simulink model "FLANFIS"  (R2017b)
settings: Solver=FixedStepAuto  StartTime=0.0  StopTime=0.1  MaxStep=1e-4  RelTol=1e-3
libraries: powerlib x86, fl_lib x45, nesl_utility x9, powerlib_meascontrol x9, elec_lib x8, fuzblock x2, simulink x2
settings Model: Creator=wolfm  LastModifiedBy=wolfm

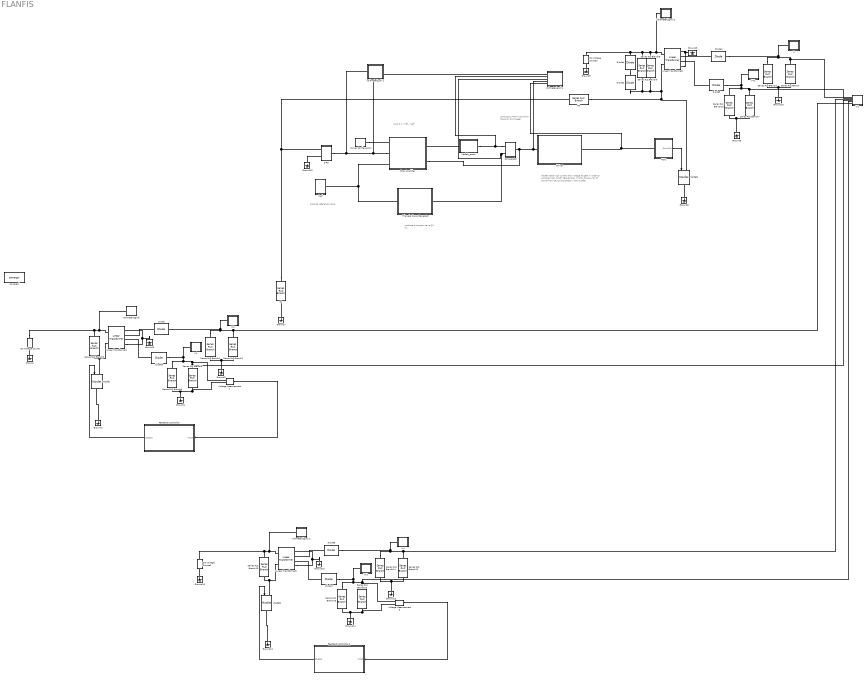
== system FLANFIS ==
  note: produces a PWM wave from the error and trigger
  note: Vout = A *( FB - Vref )
  note: produce a triangle wave @ f Hz
  note: produce reference Value
  note: Mosfet need high current and voltage at gate in order to produce high switch frequencies. IT also saves a lot of power from being dissipated in the mosfet.
  "Comparator " : Subsystem
  DC Voltage Source : powerlib/Electrical Sources/DC Voltage Source  Amplitude=24  Measurements=None
  DC Voltage Source1 : powerlib/Electrical Sources/DC Voltage Source  Amplitude=24  Measurements=None
  DC Voltage Source2 : powerlib/Electrical Sources/DC Voltage Source  Amplitude=24  Measurements=None
  Diode{,1..3,5..7} (7 alike) : powerlib/Power Electronics/Diode  Ron=0.001  Lon=0  Vf=0.7  IC=0  UseSnubber=0  Rs=500  Cs=250e-9  Measurements=off
  Diode4 : powerlib/Power Electronics/Diode  Ron=0.001  Lon=0  Vf=5.7  IC=0  UseSnubber=0  Rs=500  Cs=250e-9  Measurements=off
  Driver : Subsystem
  Error Amplifier : Subsystem
  "Feedback Controller " : Subsystem
  Feedback Controller 2 : Subsystem
  Ground{,1..16} (17 alike) : powerlib/Elements/Ground  LConnTagsString=a
  Linear Transformer1 : powerlib/Elements/Linear Transformer  UNITS=SI  NominalPower=[ 250e6 60 ]  winding1=[7.35e+05 4.3218 0.8]  winding2="[7.35e+05  4.3218 0.8]"  ThreeWindings=on  winding3=[7.35e+05 4.3218 0.8]  RmLm=[1.0805e+06 2880]  Measurements=None  DataType=on
  Linear Transformer2 : powerlib/Elements/Linear Transformer  UNITS=SI  NominalPower=[ 250e6 60 ]  winding1=[7.35e+05 4.3218 0.8]  winding2=[7.35e+05*15.5/24 4.3218 0.8]  ThreeWindings=on  winding3=[7.35e+05*15.5/24 4.3218 0.8]  RmLm=[1.0805e+06 2880]  Measurements=None  DataType=on
  Linear Transformer3 : powerlib/Elements/Linear Transformer  UNITS=SI  NominalPower=[ 250e6 60 ]  winding1=[7.35e+05 4.3218 0.8]  winding2="[7.35e+05  4.3218 0.8]"  ThreeWindings=on  winding3=[7.35e+05 4.3218 0.8]  RmLm=[1.0805e+06 2880]  Measurements=None  DataType=on
  Matlab_errors : Subsystem
  Mosfet : powerlib/Power Electronics/Mosfet  Ron=0.1  Lon=0  Rd=0.01  Vfd=0.7  IC=0  Rs=1e5  Cs=inf  Measurements=off
  Mosfet1 : powerlib/Power Electronics/Mosfet  Ron=0.1  Lon=0  Rd=0.01  Vfd=0.7  IC=0  Rs=1e5  Cs=inf  Measurements=off
  Mosfet2 : powerlib/Power Electronics/Mosfet  Ron=0.1  Lon=0  Rd=0.01  Vfd=0.7  IC=0  Rs=1e5  Cs=inf  Measurements=off
  PS-S : Subsystem
  R1 : powerlib/Elements/Series RLC Branch  LConnTagsString=__new0  RConnTagsString=__new0  BranchType=R  Resistance=3.9e+3  Inductance=0  SetiL0=off  InitialCurrent=0  Capacitance=0  Setx0=off  InitialVoltage=0  Measurements=None
  R5 : powerlib/Elements/Series RLC Branch  LConnTagsString=__new0  RConnTagsString=__new0  BranchType=R  Resistance=76.8e+3  Inductance=0  SetiL0=off  InitialCurrent=0  Capacitance=0  Setx0=off  InitialVoltage=0  Measurements=None
  S-PS : Subsystem
  Series RLC Branch{,2,5,7,12,15} (6 alike) : powerlib/Elements/Series RLC Branch  LConnTagsString=__new0  RConnTagsString=__new0  BranchType=R  Resistance=4.7e+3  Inductance=0  SetiL0=off  InitialCurrent=0  Capacitance=0  Setx0=off  InitialVoltage=0  Measurements=None
  Series RLC Branch{1,4,6,10,14,16} (6 alike) : powerlib/Elements/Series RLC Branch  LConnTagsString=__new0  RConnTagsString=__new0  BranchType=C  Resistance=15  Inductance=0  SetiL0=off  InitialCurrent=0  Capacitance=10e-6  Setx0=off  InitialVoltage=0  Measurements=None
  Series RLC Branch13 : powerlib/Elements/Series RLC Branch  LConnTagsString=__new0  RConnTagsString=__new0  BranchType=RC  Resistance=1e+3  Inductance=0  SetiL0=off  InitialCurrent=0  Capacitance=4.6e-7  Setx0=off  InitialVoltage=0  Measurements=None
  Series RLC Branch3 : powerlib/Elements/Series RLC Branch  LConnTagsString=__new0  RConnTagsString=__new0  BranchType=RC  Resistance=1e+3  Inductance=0  SetiL0=off  InitialCurrent=0  Capacitance=4.6e-6  Setx0=off  InitialVoltage=0  Measurements=None
  Series RLC Branch8 : powerlib/Elements/Series RLC Branch  LConnTagsString=__new0  RConnTagsString=__new0  BranchType=RC  Resistance=1e+3  Inductance=0  SetiL0=off  InitialCurrent=0  Capacitance=4.6e-6  Setx0=off  InitialVoltage=0  Measurements=None
  Series RLC Branch9 : powerlib/Elements/Series RLC Branch  LConnTagsString=__new0  RConnTagsString=__new0  BranchType=C  Resistance=15  Inductance=0  SetiL0=off  InitialCurrent=0  Capacitance=5.7e-6  Setx0=off  InitialVoltage=0  Measurements=None
  Solver Configuration : nesl_utility/Solver Configuration  PhysicalDomain=network_engine_domain  SubClassName=solver  LeftPortType=input  RightPortType=generic  Accelerate=off  Tones=[]  Harmonics=[]  SimulateNoise=off  Profile=off  UseLocalSampling=off  EnableSwitchedLinearOptims=on  FrequencyDomain=off  UseCCode=off  RelTol=0.001  AbsTol=1e-06  MinStep=1e-09  ToWorkspace=off  RevertToSquareIcSolve=off  NumHomotopyIterations=100  PhasorMode=off  PhasorModeNumHarmonics=1  DoDC=off  ResidualTolerance=1e-09  UseLocalSolver=off  LocalSolverChoice=NE_BACKWARD_EULER_ADVANCER  LocalSolverSampleTime=0.001  DoFixedCost=off  MaxNonlinIter=3  MaxModeIter=2  LinearAlgebra=Sparse  DelaysMemoryBudget=1024  AutomaticFiltering=on  FilteringTimeConstant=0.001
  Triangle Wave Generator : Subsystem
  V+ : Subsystem
  V+1 : Subsystem
  V+2 : Subsystem
  V- : Subsystem
  V-1 : Subsystem
  V-2 : Subsystem
  V-4 : Subsystem
  Voltage Measurement1 : powerlib/Measurements/Voltage Measurement  PhasorSimulation=off  OutputType=Complex  PSBequivalent=0
  Voltage Measurement3 : powerlib/Measurements/Voltage Measurement  PhasorSimulation=off  OutputType=Complex  PSBequivalent=0
  "Voltmeter(Sgnd) " : Subsystem
  Voltmeter(Sgnd) 1 : Subsystem
  Voltmeter(Sgnd) 2 : Subsystem
  Voltmeter(gnd) 1 : Subsystem
  Voltmeter(gnd) 4 : Subsystem
  Vref : Subsystem
  powergui : powerlib/powergui  Priority=1  SimulationMode=Discrete  SampleTime=50e-6  frequency=60  Iterations=50  frequencyindice=0  Pbase=100e6  ErrMax=1e-4  UnitsV=kV  UnitsW=MW  buscounter=0  FunctionMessages=off  echomessages=off  EnableUseOfTLC=off  CurrentSourceSwitches=off  DisableSnubberDevices=off  DisableRonSwitches=off  DisableVfSwitches=off  DisplayEquations=off  SolverType=Tustin/Backward Euler (TBE)  Interpol=off  ExternalGateDelay=off  methode=off  Ts=100  x0status=blocks  SPID=off  SwTol=0  HookPort=off  RestoreLinks=warning  ResistiveCurrentMeasurement=off  Frange=[0:2:500]  Ylog=off  Xlog=on  ShowGrid=off  save=off  variable=ZData  structure=0  ZoomFFT=off  StartTime=0.0  cycles=1  DisplayStyle=1  fundamental=60  FreqAxis=off  MaxFrequency=1000  frequencyindicesteady=1  RmsSteady=1  display=off
  wires:
  Voltage Measurement1/1 -> "Feedback Controller "/1("Input ")
  "Feedback Controller "/1("Output ") -> Mosfet/1
  Feedback Controller 2/1("Output ") -> Mosfet2/1
  Voltage Measurement3/1 -> Feedback Controller 2/1("Input ")
  PS-S/1("Simulink ") -> Mosfet1/1
  connections:
  Linear Transformer1/LConn2 -- Mosfet/LConn1 -- Series RLC Branch3/LConn1
  DC Voltage Source/RConn1 -- Series RLC Branch3/RConn1 -- Linear Transformer1/LConn1 -- "Voltmeter(Sgnd) "/LConn1
  Ground/LConn1 -- DC Voltage Source/LConn1
  Ground1/LConn1 -- Mosfet/RConn1
  Ground4/LConn1 -- Voltage Measurement1/LConn2 -- Series RLC Branch5/LConn1 -- Series RLC Branch6/LConn1
  Series RLC Branch5/RConn1 -- V-2/LConn4 -- Series RLC Branch6/RConn1 -- V+/LConn1 -- Diode3/RConn1 -- Voltage Measurement1/LConn1
  Series RLC Branch2/LConn1 -- Series RLC Branch4/LConn1 -- Ground2/LConn1
  Series RLC Branch4/RConn1 -- V-2/LConn6 -- Series RLC Branch2/RConn1 -- V-1/LConn1 -- Diode/LConn1
  Diode/RConn1 -- Linear Transformer1/RConn2
  Diode3/LConn1 -- Linear Transformer1/RConn3
  Linear Transformer1/RConn4 -- Ground3/LConn1 -- Linear Transformer1/RConn1
  Series RLC Branch13/LConn1 -- Linear Transformer3/LConn2 -- Mosfet2/LConn1
  Linear Transformer3/RConn1 -- Linear Transformer3/RConn4 -- Ground13/LConn1
  Series RLC Branch16/RConn1 -- Series RLC Branch15/RConn1 -- Voltage Measurement3/LConn1 -- V-2/LConn5 -- V+2/LConn1 -- Diode7/RConn1
  Series RLC Branch14/RConn1 -- Series RLC Branch12/RConn1 -- V-2/LConn3 -- V-4/LConn1 -- Diode6/LConn1
  Series RLC Branch16/LConn1 -- Ground14/LConn1 -- Voltage Measurement3/LConn2 -- Series RLC Branch15/LConn1
  Ground12/LConn1 -- Series RLC Branch12/LConn1 -- Series RLC Branch14/LConn1
  Voltmeter(Sgnd) 2/LConn1 -- Linear Transformer3/LConn1 -- DC Voltage Source2/RConn1 -- Series RLC Branch13/RConn1
  Ground11/LConn1 -- Mosfet2/RConn1
  Diode6/RConn1 -- Linear Transformer3/RConn2
  Ground10/LConn1 -- DC Voltage Source2/LConn1
  Diode7/LConn1 -- Linear Transformer3/RConn3
  Error Amplifier/LConn2 -- S-PS/RConn1 -- Voltmeter(gnd) 1/LConn1 -- Voltmeter(gnd) 4/LConn1
  Linear Transformer2/RConn1 -- Linear Transformer2/RConn4 -- Ground8/LConn1
  Driver/LConn1 -- Voltmeter(gnd) 4/LConn4 -- "Comparator "/RConn1 -- Error Amplifier/RConn2
  Series RLC Branch1/RConn1 -- V-2/LConn1 -- Series RLC Branch/RConn1 -- V-/LConn1 -- Diode1/LConn1
  R1/RConn1 -- R5/LConn1 -- S-PS/LConn1
  Series RLC Branch7/RConn1 -- V-2/LConn2 -- Series RLC Branch10/RConn1 -- V+1/LConn1 -- Diode5/RConn1
  Series RLC Branch10/LConn1 -- Series RLC Branch7/LConn1 -- Ground9/LConn1
  Voltmeter(gnd) 4/LConn5 -- PS-S/LConn1 -- Driver/RConn1
  R5/RConn1 -- Mosfet1/LConn1 -- Series RLC Branch8/LConn1 -- Series RLC Branch9/LConn1 -- Diode2/LConn1 -- Linear Transformer2/LConn2
  Vref/LConn1 -- Triangle Wave Generator/LConn1 -- Error Amplifier/LConn3
  Triangle Wave Generator/RConn1 -- "Comparator "/LConn2 -- Voltmeter(gnd) 4/LConn3
  Series RLC Branch9/RConn1 -- DC Voltage Source1/RConn1 -- Diode4/LConn1 -- Series RLC Branch8/RConn1 -- Linear Transformer2/LConn1 -- Voltmeter(Sgnd) 1/LConn1
  Series RLC Branch/LConn1 -- Series RLC Branch1/LConn1 -- Ground16/LConn1
  "Comparator "/LConn1 -- Matlab_errors/RConn1 -- Voltmeter(gnd) 4/LConn2
  Ground15/LConn1 -- S-PS/LConn2
  Ground5/LConn1 -- DC Voltage Source1/LConn1
  Ground6/LConn1 -- Mosfet1/RConn1
  Solver Configuration/RConn1 -- Error Amplifier/LConn1
  Diode4/RConn1 -- Diode2/RConn1
  Ground7/LConn1 -- R1/LConn1
  Matlab_errors/LConn1 -- Error Amplifier/RConn1
  Diode5/LConn1 -- Linear Transformer2/RConn3
  Diode1/RConn1 -- Linear Transformer2/RConn2

== system FLANFIS/Comparator  ==
  Comparator : elec_lib/Integrated Circuits/Comparator  V_OS=5 mV  V_OL=0 V  V_OH=5 V  C_IN=0 pF  R_OUT=2 Ohm  Delay=0 s
      settings: SourceProductName=Simscape Electronics  SourceProductBaseCode=SN
  Vin1 : PMIOPort  Port=1  Side=Left
  Output : PMIOPort  Port=2  Side=Right
  VIn2 : PMIOPort  Port=3  Side=Left
  connections:
  Vin1/RConn1 -- Comparator/LConn1
  Comparator/LConn2 -- VIn2/RConn1
  Comparator/RConn1 -- Output/RConn1

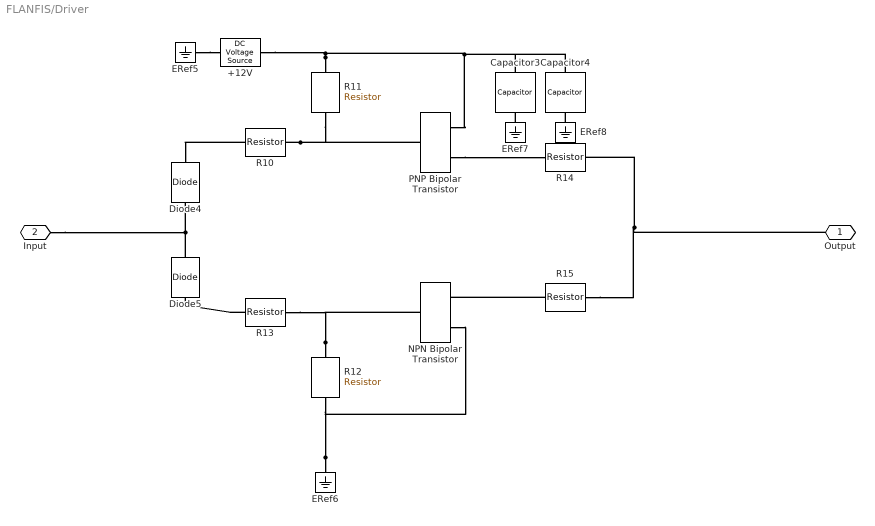
== system FLANFIS/Driver ==
  "+12V " : elec_lib/Additional Components/SPICE-Compatible Components/Sources/DC Voltage Source  DC=12 V
      settings: SourceProductName=Simscape Electronics  SourceProductBaseCode=SN
  Capacitor3 : fl_lib/Electrical/Electrical Elements/Capacitor  c=47e-6 F  r=0 Ohm  g=0 1/Ohm  i_specify=off  i_priority=None  i=0 A  i_nominal_specify=off  i_nominal_unit=A  i_nominal_value=1  v_specify=off  v_priority=None  v=0 V  v_nominal_specify=off  v_nominal_unit=V  v_nominal_value=1  vc_specify=off  vc_priority=High  vc=0 V  vc_nominal_specify=off  vc_nominal_unit=V  vc_nominal_value=1
  Capacitor4 : fl_lib/Electrical/Electrical Elements/Capacitor  c=100e-9 F  r=0 Ohm  g=0 1/Ohm  i_specify=off  i_priority=None  i=0 A  i_nominal_specify=off  i_nominal_unit=A  i_nominal_value=1  v_specify=off  v_priority=None  v=0 V  v_nominal_specify=off  v_nominal_unit=V  v_nominal_value=1  vc_specify=off  vc_priority=High  vc=0 V  vc_nominal_specify=off  vc_nominal_unit=V  vc_nominal_value=1
  Diode4 : elec_lib/Semiconductor Devices/Diode  ModelType=2  Vf=3.3 V  Ron=0.3 Ohm  Goff=1e-8 S  Rz=0.3 Ohm  Vz=50 V  C_PWL=5 pF  prmExp=1  I12=[.0137, .545] A  V12=[.6, .7] V  I1=0.0137 A  V1=0.6 V  IS=1e-12 A  ec=1  RS=0.01 Ohm  Tmeas=25 degC  BV=inf V  C_param=1  CJ0=5 pF  VJ=1 V  Mgrad=0.5  Vvec=[.1, 10, 100] V  Cvec=[3.5, 1, .4] pF  FC=0.5  Q_param=1  Irrm=-7.15 A  iF=4 A  didt=-750 A/us  trr=115 ns  TT=50 ns  tau=100 ns  T_param=1  IS_T2=1.25e-7 A  I1_T2=0.245 A  V1_T2=0.5 V  Tmeas2=125 degC  EG_param=1  EG=1.11 eV  XTI_param=1  XTI=3  dBVdT=0 V/K  Tdevice=25 degC  i_capacitor_specify=off  i_capacitor_priority=High  i_capacitor=0 A  i_capacitor_nominal_specify=off  i_capacitor_nominal_unit=A  i_capacitor_nominal_value=1  v_capacitor_specify=off  v_capacitor_priority=None  v_capacitor=0 V  v_capacitor_nominal_specify=off  v_capacitor_nominal_unit=V  v_capacitor_nominal_value=1  Rth=[0, 10] K/W  thermal_mass_parameterization=1  thermal_mass=[0, 1] J/K  thermal_time_constant=[0, 10] s  thermal_mass_initial_temperatures=[25, 25] degC
      settings: SourceProductName=Simscape Electronics  SourceProductBaseCode=SN
  Diode5 : elec_lib/Semiconductor Devices/Diode  ModelType=2  Vf=3.3 V  Ron=0.3 Ohm  Goff=1e-8 S  Rz=0.3 Ohm  Vz=50 V  C_PWL=5 pF  prmExp=1  I12=[.0137, .545] A  V12=[.6, .7] V  I1=0.0137 A  V1=0.6 V  IS=1e-12 A  ec=1  RS=0.01 Ohm  Tmeas=25 degC  BV=inf V  C_param=1  CJ0=5 pF  VJ=1 V  Mgrad=0.5  Vvec=[.1, 10, 100] V  Cvec=[3.5, 1, .4] pF  FC=0.5  Q_param=1  Irrm=-7.15 A  iF=4 A  didt=-750 A/us  trr=115 ns  TT=50 ns  tau=100 ns  T_param=1  IS_T2=1.25e-7 A  I1_T2=0.245 A  V1_T2=0.5 V  Tmeas2=125 degC  EG_param=1  EG=1.11 eV  XTI_param=1  XTI=3  dBVdT=0 V/K  Tdevice=25 degC  i_capacitor_specify=off  i_capacitor_priority=High  i_capacitor=0 A  i_capacitor_nominal_specify=off  i_capacitor_nominal_unit=A  i_capacitor_nominal_value=1  v_capacitor_specify=off  v_capacitor_priority=None  v_capacitor=0 V  v_capacitor_nominal_specify=off  v_capacitor_nominal_unit=V  v_capacitor_nominal_value=1  Rth=[0, 10] K/W  thermal_mass_parameterization=1  thermal_mass=[0, 1] J/K  thermal_time_constant=[0, 10] s  thermal_mass_initial_temperatures=[25, 25] degC
      settings: SourceProductName=Simscape Electronics  SourceProductBaseCode=SN
  ERef{5..8} (4 alike) : fl_lib/Electrical/Electrical Elements/Electrical Reference
  NPN Bipolar Transistor : elec_lib/Semiconductor Devices/NPN Bipolar Transistor  parameterization=1  prmDatasheet=1  prmEquCoeff=1  BF=100  IS=1e-14 A  ec=1  VAF=200 V  hfe=100  hoe=5e-5 1/Ohm  Ic_h=1 mA  Vce_h=5 V  V1=0.55 V  I1=0.5 mA  BR=1  Tmeas=25 degC  RC=0.01 Ohm  RE=1e-4 Ohm  RB=1 Ohm  C_BC=5 pF  C_BE=5 pF  TF=0 us  TR=0 us  hfe_T2=125  XTB=0  V1_T2=0.45 V  I1_T2=0.5 mA  Tmeas2=125 degC  EG=1.11 eV  XTI=3  TdeviceDatasheet=25 degC  TdeviceEquCoeff=25 degC  Rth=[ 0 10 ] K/W  thermal_mass_parameterization=1  thermal_mass=[ 0 1 ] J/K  thermal_time_constant=[ 0 10 ] s  thermal_mass_initial_temperatures=[ 25 25 ] degC
      settings: SourceProductName=Simscape Electronics  SourceProductBaseCode=SN
  PNP Bipolar Transistor : elec_lib/Semiconductor Devices/PNP Bipolar Transistor  parameterization=1  prmDatasheet=1  prmEquCoeff=1  BF=100  IS=1e-14 A  ec=1  VAF=200 V  hfe=100  hoe=5e-5 1/Ohm  Ic_h=-1 mA  Vce_h=-5 V  V1=-0.55 V  I1=-0.5 mA  BR=1  Tmeas=25 degC  RC=0.01 Ohm  RE=1e-4 Ohm  RB=1 Ohm  C_BC=5 pF  C_BE=5 pF  TF=0 us  TR=0 us  hfe_T2=125  XTB=0  V1_T2=-0.45 V  I1_T2=-0.5 mA  Tmeas2=125 degC  EG=1.11 eV  XTI=3  TdeviceDatasheet=25 degC  TdeviceEquCoeff=25 degC  Rth=[ 0 10 ] K/W  thermal_mass_parameterization=1  thermal_mass=[ 0 1 ] J/K  thermal_time_constant=[ 0 10 ] s  thermal_mass_initial_temperatures=[ 25 25 ] degC
      settings: SourceProductName=Simscape Electronics  SourceProductBaseCode=SN
  R10 : fl_lib/Electrical/Electrical Elements/Resistor  R=1e+3 Ohm  i_specify=off  i_priority=High  i=0 A  i_nominal_specify=off  i_nominal_unit=A  i_nominal_value=1  v_specify=off  v_priority=High  v=0 V  v_nominal_specify=off  v_nominal_unit=V  v_nominal_value=1
      settings: AttributesFormatString=%<R> %<R_unit>
  R11 : fl_lib/Electrical/Electrical Elements/Resistor  R=47e+3 Ohm  i_specify=off  i_priority=High  i=0 A  i_nominal_specify=off  i_nominal_unit=A  i_nominal_value=1  v_specify=off  v_priority=High  v=0 V  v_nominal_specify=off  v_nominal_unit=V  v_nominal_value=1
      settings: AttributesFormatString=%<R> %<R_unit>
  R12 : fl_lib/Electrical/Electrical Elements/Resistor  R=47e+3 Ohm  i_specify=off  i_priority=High  i=0 A  i_nominal_specify=off  i_nominal_unit=A  i_nominal_value=1  v_specify=off  v_priority=High  v=0 V  v_nominal_specify=off  v_nominal_unit=V  v_nominal_value=1
      settings: AttributesFormatString=%<R> %<R_unit>
  R13 : fl_lib/Electrical/Electrical Elements/Resistor  R=1e+3 Ohm  i_specify=off  i_priority=High  i=0 A  i_nominal_specify=off  i_nominal_unit=A  i_nominal_value=1  v_specify=off  v_priority=High  v=0 V  v_nominal_specify=off  v_nominal_unit=V  v_nominal_value=1
      settings: AttributesFormatString=%<R> %<R_unit>
  R14 : fl_lib/Electrical/Electrical Elements/Resistor  R=4.7 Ohm  i_specify=off  i_priority=High  i=0 A  i_nominal_specify=off  i_nominal_unit=A  i_nominal_value=1  v_specify=off  v_priority=High  v=0 V  v_nominal_specify=off  v_nominal_unit=V  v_nominal_value=1
      settings: AttributesFormatString=%<R> %<R_unit>
  R15 : fl_lib/Electrical/Electrical Elements/Resistor  R=4.7 Ohm  i_specify=off  i_priority=High  i=0 A  i_nominal_specify=off  i_nominal_unit=A  i_nominal_value=1  v_specify=off  v_priority=High  v=0 V  v_nominal_specify=off  v_nominal_unit=V  v_nominal_value=1
      settings: AttributesFormatString=%<R> %<R_unit>
  Output : PMIOPort  Port=1  Side=Right
  Input : PMIOPort  Port=2  Side=Left
  connections:
  Diode5/RConn1 -- Input/RConn1 -- Diode4/LConn1
  R15/RConn1 -- R14/LConn1 -- Output/RConn1
  ERef6/LConn1 -- R12/LConn1 -- NPN Bipolar Transistor/RConn2
  R11/RConn1 -- "+12V "/LConn1 -- Capacitor4/LConn1 -- Capacitor3/LConn1 -- PNP Bipolar Transistor/RConn1
  R12/RConn1 -- R13/LConn1 -- NPN Bipolar Transistor/LConn1
  PNP Bipolar Transistor/RConn2 -- R14/RConn1
  R15/LConn1 -- NPN Bipolar Transistor/RConn1
  R10/RConn1 -- Diode4/RConn1
  ERef5/LConn1 -- "+12V "/RConn1
  R13/RConn1 -- Diode5/LConn1
  ERef7/LConn1 -- Capacitor3/RConn1
  R10/LConn1 -- R11/LConn1 -- PNP Bipolar Transistor/LConn1
  ERef8/LConn1 -- Capacitor4/RConn1

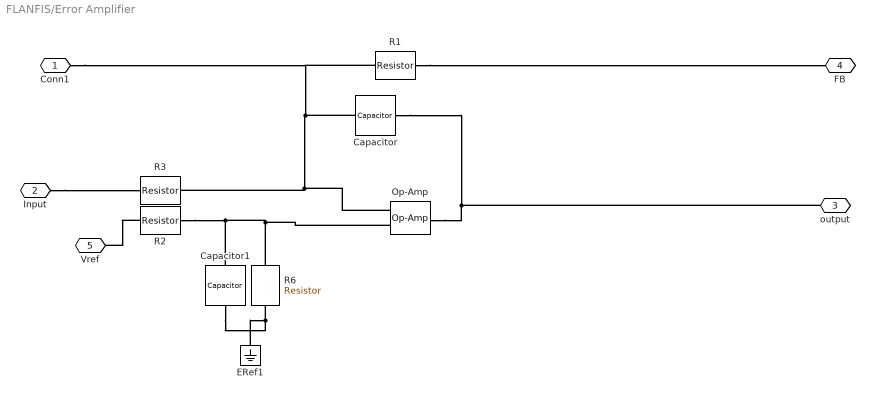
== system FLANFIS/Error Amplifier ==
  Capacitor : fl_lib/Electrical/Electrical Elements/Capacitor  c=100e-12 F  r=5 Ohm  g=0 1/Ohm  i_specify=off  i_priority=None  i=0 A  i_nominal_specify=off  i_nominal_unit=A  i_nominal_value=1  v_specify=off  v_priority=None  v=0 V  v_nominal_specify=off  v_nominal_unit=V  v_nominal_value=1  vc_specify=on  vc_priority=None  vc=0 V  vc_nominal_specify=off  vc_nominal_unit=V  vc_nominal_value=1
  Capacitor1 : fl_lib/Electrical/Electrical Elements/Capacitor  c=100e-12 F  r=0 Ohm  g=0 1/Ohm  i_specify=off  i_priority=None  i=0 A  i_nominal_specify=off  i_nominal_unit=A  i_nominal_value=1  v_specify=off  v_priority=None  v=0 V  v_nominal_specify=off  v_nominal_unit=V  v_nominal_value=1  vc_specify=off  vc_priority=High  vc=0 V  vc_nominal_specify=off  vc_nominal_unit=V  vc_nominal_value=1
  ERef1 : fl_lib/Electrical/Electrical Elements/Electrical Reference
  Op-Amp : fl_lib/Electrical/Electrical Elements/Op-Amp  outI_specify=off  outI_priority=None  outI=0 A  outI_nominal_specify=off  outI_nominal_unit=A  outI_nominal_value=1
  R{1..3,6} (4 alike) : fl_lib/Electrical/Electrical Elements/Resistor  R=10e3 Ohm  i_specify=off  i_priority=High  i=0 A  i_nominal_specify=off  i_nominal_unit=A  i_nominal_value=1  v_specify=off  v_priority=High  v=0 V  v_nominal_specify=off  v_nominal_unit=V  v_nominal_value=1
      settings: AttributesFormatString=%<R> %<R_unit>
  Conn1 : PMIOPort  Port=1  Side=Left
  Input : PMIOPort  Port=2  Side=Left
  "output " : PMIOPort  Port=3  Side=Right
  FB : PMIOPort  Port=4  Side=Right
  Vref : PMIOPort  Port=5  Side=Left
  connections:
  R1/RConn1 -- FB/RConn1
  R2/LConn1 -- Vref/RConn1
  Capacitor/LConn1 -- Op-Amp/LConn2 -- R3/RConn1 -- Conn1/RConn1 -- R1/LConn1
  R6/LConn1 -- Op-Amp/LConn1 -- R2/RConn1 -- Capacitor1/LConn1
  R6/RConn1 -- Capacitor1/RConn1 -- ERef1/LConn1
  Input/RConn1 -- R3/LConn1
  Capacitor/RConn1 -- "output "/RConn1 -- Op-Amp/RConn1

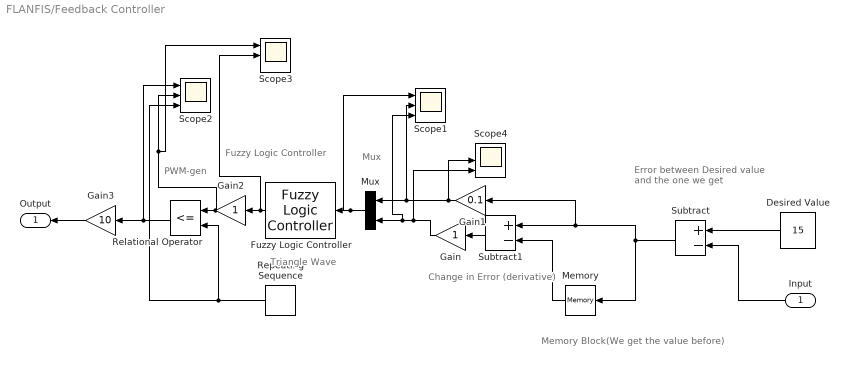
== system FLANFIS/Feedback Controller  ==
  note: PWM-gen
  note: Triangle Wave
  note: Fuzzy Logic Controller
  note: Mux
  note: Change in Error (derivative)
  note: Memory Block(We get the value before)
  note: Error between Desired value and the one we get
  "Input " : Inport
  Desired Value : Constant  Value=15
  Fuzzy Logic Controller : fuzblock/Fuzzy Logic  Controller  FIS='flc.fis'  OutputSampleNumber=1e+2  DataType=double  FuzzifiedInputs=off  RuleFiringStrengths=off  RuleOutputs=off  AggregatedOutputs=off  SimulateUsing=Interpreted execution
  Gain : Gain  OutMax=[15]
  Gain1 : Gain  Gain=0.1  OutMax=[15]
  Gain2 : Gain  OutMax=[15]
  Gain3 : Gain  Gain=10  OutMax=[15]
  Memory : Memory
  Mux : Mux  Inputs=2
  Relational Operator : RelationalOperator  Operator=<=  OutDataTypeStr=boolean  RndMeth=Simplest
  Repeating Sequence : simulink/Sources/Repeating Sequence  rep_seq_t=[0 0.5 1]/1000  rep_seq_y=[0 1 0]
  Scope{1..4} (4 alike) : Scope  NumInputPorts=3
  Subtract : Sum  Inputs=+-
  Subtract1 : Sum  Inputs=+-
  "Output " : Outport
  wires:
  Repeating Sequence/1 -> Scope2/3, Relational Operator/2
  Relational Operator/1 -> Scope2/1, Gain3/1
  Mux/1 -> Scope1/1, Fuzzy Logic Controller/1
  Subtract/1 -> Memory/1, Gain1/1, Subtract1/1
  Desired Value/1 -> Subtract/1
  "Input "/1 -> Subtract/2
  Memory/1 -> Subtract1/2
  Subtract1/1 -> Gain/1
  Gain/1 -> Scope4/3, Scope1/3, Mux/2
  Gain1/1 -> Scope4/2, Scope1/2, Mux/1
  Gain2/1 -> Scope3/1, Scope2/2, Relational Operator/1
  Fuzzy Logic Controller/1 -> Scope3/2, Gain2/1
  Gain3/1 -> "Output "/1

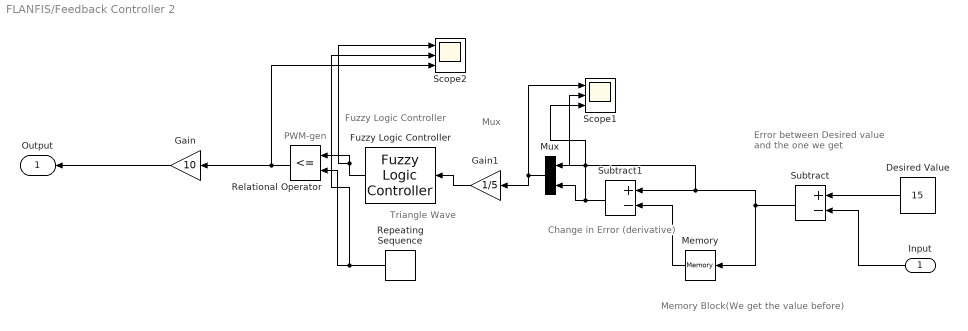
== system FLANFIS/Feedback Controller 2 ==
  note: PWM-gen
  note: Triangle Wave
  note: Fuzzy Logic Controller
  note: Mux
  note: Change in Error (derivative)
  note: Memory Block(We get the value before)
  note: Error between Desired value and the one we get
  "Input " : Inport
  Desired Value : Constant  Value=15
  Fuzzy Logic Controller : fuzblock/Fuzzy Logic  Controller  FIS='flc.fis'  OutputSampleNumber=101  DataType=double  FuzzifiedInputs=off  RuleFiringStrengths=off  RuleOutputs=off  AggregatedOutputs=off  SimulateUsing=Interpreted execution
  Gain : Gain  Gain=10
  Gain1 : Gain  Gain=1/5
  Memory : Memory
  Mux : Mux  Inputs=2
  Relational Operator : RelationalOperator  Operator=<=  OutDataTypeStr=boolean  RndMeth=Simplest
  Repeating Sequence : simulink/Sources/Repeating Sequence  rep_seq_t=[0 0.5 1]/500  rep_seq_y=[0 15 0]
  Scope1 : Scope  NumInputPorts=3
  Scope2 : Scope  NumInputPorts=3
  Subtract : Sum  Inputs=+-
  Subtract1 : Sum  Inputs=+-
  "Output " : Outport
  wires:
  Subtract1/1 -> Scope1/2, Scope1/3, Mux/2
  Repeating Sequence/1 -> Scope2/2, Relational Operator/2
  Relational Operator/1 -> Scope2/3, Gain/1
  Subtract/1 -> Memory/1, Mux/1, Subtract1/1
  Desired Value/1 -> Subtract/1
  "Input "/1 -> Subtract/2
  Memory/1 -> Subtract1/2
  Fuzzy Logic Controller/1 -> Scope2/1, Relational Operator/1
  Gain/1 -> "Output "/1
  Mux/1 -> Scope1/1, Gain1/1
  Gain1/1 -> Fuzzy Logic Controller/1

== system FLANFIS/Matlab_errors ==
  Capacitor5 : fl_lib/Electrical/Electrical Elements/Capacitor  c=100e-6 F  r=10 Ohm  g=0 1/Ohm  i_specify=off  i_priority=None  i=0 A  i_nominal_specify=off  i_nominal_unit=A  i_nominal_value=1  v_specify=off  v_priority=None  v=0 V  v_nominal_specify=off  v_nominal_unit=V  v_nominal_value=1  vc_specify=on  vc_priority=None  vc=0 V  vc_nominal_specify=off  vc_nominal_unit=V  vc_nominal_value=1
  ERef4 : fl_lib/Electrical/Electrical Elements/Electrical Reference
  R7 : fl_lib/Electrical/Electrical Elements/Resistor  R=10e5 Ohm  i_specify=off  i_priority=High  i=0 A  i_nominal_specify=off  i_nominal_unit=A  i_nominal_value=1  v_specify=off  v_priority=High  v=0 V  v_nominal_specify=off  v_nominal_unit=V  v_nominal_value=1
      settings: AttributesFormatString=%<R> %<R_unit>
  Output : PMIOPort  Port=1  Side=Right
  "Input " : PMIOPort  Port=2  Side=Left
  connections:
  R7/LConn1 -- "Input "/RConn1
  ERef4/LConn1 -- Capacitor5/RConn1
  R7/RConn1 -- Output/RConn1 -- Capacitor5/LConn1

== system FLANFIS/PS-S ==
  ERef9 : fl_lib/Electrical/Electrical Elements/Electrical Reference
  PS-Simulink Converter1 : nesl_utility/PS-Simulink Converter  PhysicalDomain=network_engine_domain  SubClassName=ps_output  LeftPortType=input  RightPortType=output  PseudoPeriodic=off  Frequencies=[]  Unit=1  AffineConversion=off
  Voltage Sensor : fl_lib/Electrical/Electrical Sensors/Voltage Sensor
  V+ : PMIOPort  Port=1  Side=Left
  "Simulink " : Outport
  wires:
  PS-Simulink Converter1/1 -> "Simulink "/1
  connections:
  Voltage Sensor/LConn1 -- V+/RConn1
  Voltage Sensor/RConn1 -- PS-Simulink Converter1/LConn1
  Voltage Sensor/RConn2 -- ERef9/LConn1

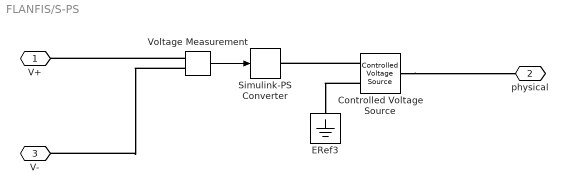
== system FLANFIS/S-PS ==
  Controlled Voltage Source : fl_lib/Electrical/Electrical Sources/Controlled Voltage Source
  ERef3 : fl_lib/Electrical/Electrical Elements/Electrical Reference
  Simulink-PS Converter : nesl_utility/Simulink-PS Converter  PhysicalDomain=network_engine_domain  SubClassName=ps_input  LeftPortType=input  RightPortType=output  PseudoPeriodic=off  Frequencies=[]  NoiseDistribution=none  NoiseParameters=[]  Unit=1  AffineConversion=off  FilteringAndDerivatives=provide  SimscapeFilterOrder=1  InputFilterTimeConstant=0.001  UdotUserProvided=0
  Voltage Measurement : powerlib/Measurements/Voltage Measurement  PhasorSimulation=off  OutputType=Complex  PSBequivalent=0
  V+ : PMIOPort  Port=1  Side=Left
  physical : PMIOPort  Port=2  Side=Right
  V- : PMIOPort  Port=3  Side=Left
  wires:
  Voltage Measurement/1 -> Simulink-PS Converter/1
  connections:
  Voltage Measurement/LConn2 -- V-/RConn1
  Voltage Measurement/LConn1 -- V+/RConn1
  Controlled Voltage Source/RConn2 -- ERef3/LConn1
  Controlled Voltage Source/RConn1 -- Simulink-PS Converter/RConn1
  Controlled Voltage Source/LConn1 -- physical/RConn1

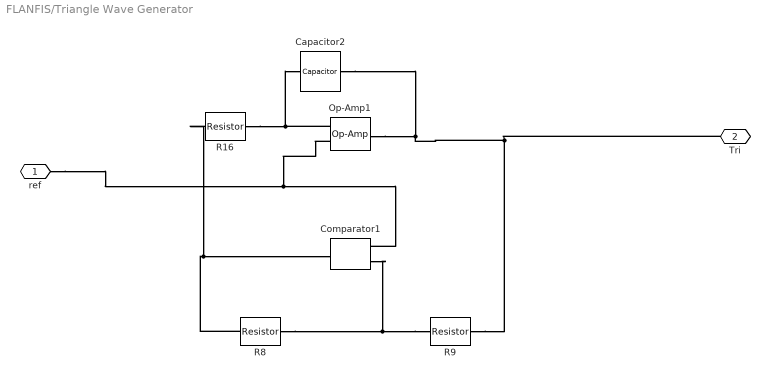
== system FLANFIS/Triangle Wave Generator ==
  Capacitor2 : fl_lib/Electrical/Electrical Elements/Capacitor  c=50e-10 F  r=2 Ohm  g=0 1/Ohm  i_specify=off  i_priority=None  i=0 A  i_nominal_specify=off  i_nominal_unit=A  i_nominal_value=1  v_specify=off  v_priority=None  v=0 V  v_nominal_specify=off  v_nominal_unit=V  v_nominal_value=1  vc_specify=off  vc_priority=High  vc=0 V  vc_nominal_specify=off  vc_nominal_unit=V  vc_nominal_value=1
  Comparator1 : elec_lib/Integrated Circuits/Comparator  V_OS=5 mV  V_OL=0 V  V_OH=6 V  C_IN=0 pF  R_OUT=1 Ohm  Delay=0 s
      settings: SourceProductName=Simscape Electronics  SourceProductBaseCode=SN
  Op-Amp1 : fl_lib/Electrical/Electrical Elements/Op-Amp  outI_specify=off  outI_priority=None  outI=0 A  outI_nominal_specify=off  outI_nominal_unit=A  outI_nominal_value=1
  R16 : fl_lib/Electrical/Electrical Elements/Resistor  R=5.9e3 Ohm  i_specify=off  i_priority=High  i=0 A  i_nominal_specify=off  i_nominal_unit=A  i_nominal_value=1  v_specify=off  v_priority=High  v=0 V  v_nominal_specify=off  v_nominal_unit=V  v_nominal_value=1
      settings: AttributesFormatString=%<R> %<R_unit>
  R8 : fl_lib/Electrical/Electrical Elements/Resistor  R=10e3 Ohm  i_specify=off  i_priority=High  i=0 A  i_nominal_specify=off  i_nominal_unit=A  i_nominal_value=1  v_specify=off  v_priority=High  v=0 V  v_nominal_specify=off  v_nominal_unit=V  v_nominal_value=1
      settings: AttributesFormatString=%<R> %<R_unit>
  R9 : fl_lib/Electrical/Electrical Elements/Resistor  R=8.45e+3 Ohm  i_specify=off  i_priority=High  i=0 A  i_nominal_specify=off  i_nominal_unit=A  i_nominal_value=1  v_specify=off  v_priority=High  v=0 V  v_nominal_specify=off  v_nominal_unit=V  v_nominal_value=1
      settings: AttributesFormatString=%<R> %<R_unit>
  ref : PMIOPort  Port=1  Side=Left
  Tri : PMIOPort  Port=2  Side=Right
  connections:
  R9/LConn1 -- Tri/RConn1 -- Op-Amp1/RConn1 -- Capacitor2/LConn1
  Comparator1/LConn2 -- ref/RConn1 -- Op-Amp1/LConn1
  R8/RConn1 -- R16/RConn1 -- Comparator1/RConn1
  Capacitor2/RConn1 -- Op-Amp1/LConn2 -- R16/LConn1
  R9/RConn1 -- R8/LConn1 -- Comparator1/LConn1

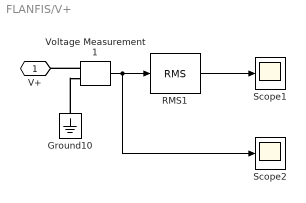
== system FLANFIS/V+ ==
  Ground10 : powerlib/Elements/Ground  LConnTagsString=a
  RMS1 : powerlib_meascontrol/Measurements/RMS  TrueRMS=on  Freq=50  RMSInit=0  Ts=1e-4
  Scope1 : Scope
  Scope2 : Scope
  Voltage Measurement1 : powerlib/Measurements/Voltage Measurement  PhasorSimulation=off  OutputType=Complex  PSBequivalent=0
  V+ : PMIOPort  Port=1  Side=Left
  wires:
  RMS1/1 -> Scope1/1
  Voltage Measurement1/1 -> RMS1/1, Scope2/1
  connections:
  Ground10/LConn1 -- Voltage Measurement1/LConn2
  Voltage Measurement1/LConn1 -- V+/RConn1

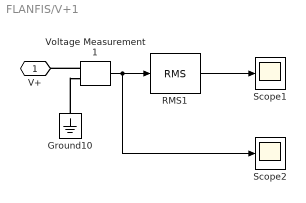
== system FLANFIS/V+1 ==
  Ground10 : powerlib/Elements/Ground  LConnTagsString=a
  RMS1 : powerlib_meascontrol/Measurements/RMS  TrueRMS=on  Freq=50  RMSInit=0  Ts=1e-4
  Scope1 : Scope
  Scope2 : Scope
  Voltage Measurement1 : powerlib/Measurements/Voltage Measurement  PhasorSimulation=off  OutputType=Complex  PSBequivalent=0
  V+ : PMIOPort  Port=1  Side=Left
  wires:
  RMS1/1 -> Scope1/1
  Voltage Measurement1/1 -> RMS1/1, Scope2/1
  connections:
  Ground10/LConn1 -- Voltage Measurement1/LConn2
  Voltage Measurement1/LConn1 -- V+/RConn1

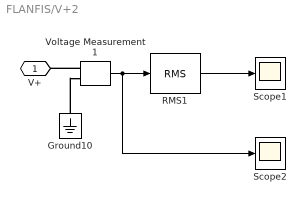
== system FLANFIS/V+2 ==
  Ground10 : powerlib/Elements/Ground  LConnTagsString=a
  RMS1 : powerlib_meascontrol/Measurements/RMS  TrueRMS=on  Freq=50  RMSInit=0  Ts=1e-4
  Scope1 : Scope
  Scope2 : Scope
  Voltage Measurement1 : powerlib/Measurements/Voltage Measurement  PhasorSimulation=off  OutputType=Complex  PSBequivalent=0
  V+ : PMIOPort  Port=1  Side=Left
  wires:
  RMS1/1 -> Scope1/1
  Voltage Measurement1/1 -> RMS1/1, Scope2/1
  connections:
  Ground10/LConn1 -- Voltage Measurement1/LConn2
  Voltage Measurement1/LConn1 -- V+/RConn1

== system FLANFIS/V- ==
  Ground10 : powerlib/Elements/Ground  LConnTagsString=a
  RMS1 : powerlib_meascontrol/Measurements/RMS  TrueRMS=on  Freq=50  RMSInit=0  Ts=1e-4
  Scope1 : Scope
  Scope2 : Scope
  Voltage Measurement1 : powerlib/Measurements/Voltage Measurement  PhasorSimulation=off  OutputType=Complex  PSBequivalent=0
  V+ : PMIOPort  Port=1  Side=Left
  wires:
  Voltage Measurement1/1 -> Scope2/1, RMS1/1
  RMS1/1 -> Scope1/1
  connections:
  Voltage Measurement1/LConn1 -- V+/RConn1
  Ground10/LConn1 -- Voltage Measurement1/LConn2

== system FLANFIS/V-1 ==
  Ground10 : powerlib/Elements/Ground  LConnTagsString=a
  RMS1 : powerlib_meascontrol/Measurements/RMS  TrueRMS=on  Freq=50  RMSInit=0  Ts=1e-4
  Scope1 : Scope
  Scope2 : Scope
  Voltage Measurement1 : powerlib/Measurements/Voltage Measurement  PhasorSimulation=off  OutputType=Complex  PSBequivalent=0
  V+ : PMIOPort  Port=1  Side=Left
  wires:
  Voltage Measurement1/1 -> Scope2/1, RMS1/1
  RMS1/1 -> Scope1/1
  connections:
  Voltage Measurement1/LConn1 -- V+/RConn1
  Ground10/LConn1 -- Voltage Measurement1/LConn2

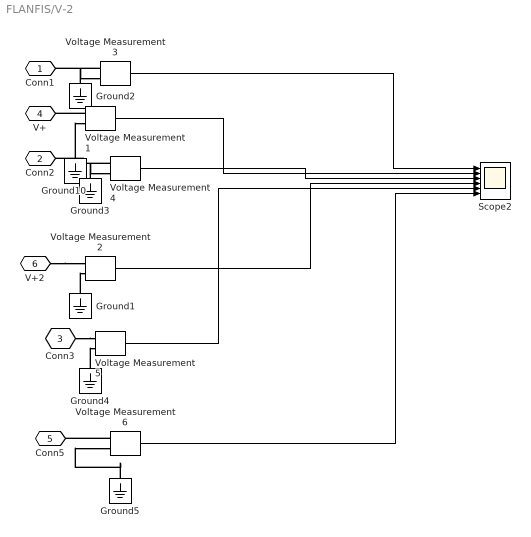
== system FLANFIS/V-2 ==
  Ground{1..5,10} (6 alike) : powerlib/Elements/Ground  LConnTagsString=a
  Scope2 : Scope  NumInputPorts=6
  Voltage Measurement{1..6} (6 alike) : powerlib/Measurements/Voltage Measurement  PhasorSimulation=off  OutputType=Complex  PSBequivalent=0
  Conn1 : PMIOPort  Port=1  Side=Left
  Conn2 : PMIOPort  Port=2  Side=Left
  Conn3 : PMIOPort  Port=3  Side=Left
  V+ : PMIOPort  Port=4  Side=Left
  Conn5 : PMIOPort  Port=5  Side=Left
  V+2 : PMIOPort  Port=6  Side=Left
  wires:
  Voltage Measurement1/1 -> Scope2/2
  Voltage Measurement2/1 -> Scope2/4
  Voltage Measurement3/1 -> Scope2/1
  Voltage Measurement4/1 -> Scope2/3
  Voltage Measurement5/1 -> Scope2/5
  Voltage Measurement6/1 -> Scope2/6
  connections:
  Ground10/LConn1 -- Voltage Measurement1/LConn2
  Voltage Measurement1/LConn1 -- V+/RConn1
  V+2/RConn1 -- Voltage Measurement2/LConn1
  Ground1/LConn1 -- Voltage Measurement2/LConn2
  Voltage Measurement3/LConn1 -- Conn1/RConn1
  Ground2/LConn1 -- Voltage Measurement3/LConn2
  Ground3/LConn1 -- Voltage Measurement4/LConn2
  Voltage Measurement4/LConn1 -- Conn2/RConn1
  Ground4/LConn1 -- Voltage Measurement5/LConn2
  Conn3/RConn1 -- Voltage Measurement5/LConn1
  Voltage Measurement6/LConn1 -- Conn5/RConn1
  Ground5/LConn1 -- Voltage Measurement6/LConn2

== system FLANFIS/V-4 ==
  Ground10 : powerlib/Elements/Ground  LConnTagsString=a
  RMS1 : powerlib_meascontrol/Measurements/RMS  TrueRMS=on  Freq=50  RMSInit=0  Ts=1e-4
  Scope1 : Scope
  Scope2 : Scope
  Voltage Measurement1 : powerlib/Measurements/Voltage Measurement  PhasorSimulation=off  OutputType=Complex  PSBequivalent=0
  V+ : PMIOPort  Port=1  Side=Left
  wires:
  Voltage Measurement1/1 -> Scope2/1, RMS1/1
  RMS1/1 -> Scope1/1
  connections:
  Voltage Measurement1/LConn1 -- V+/RConn1
  Ground10/LConn1 -- Voltage Measurement1/LConn2

== system FLANFIS/Voltmeter(Sgnd)  ==
  Ground10 : powerlib/Elements/Ground  LConnTagsString=a
  RMS1 : powerlib_meascontrol/Measurements/RMS  TrueRMS=on  Freq=50  RMSInit=0  Ts=1e-4
  Scope1 : Scope
  Scope2 : Scope
  Voltage Measurement1 : powerlib/Measurements/Voltage Measurement  PhasorSimulation=off  OutputType=Complex  PSBequivalent=0
  V+ : PMIOPort  Port=1  Side=Left
  wires:
  Voltage Measurement1/1 -> Scope2/1, RMS1/1
  RMS1/1 -> Scope1/1
  connections:
  Voltage Measurement1/LConn1 -- V+/RConn1
  Ground10/LConn1 -- Voltage Measurement1/LConn2

== system FLANFIS/Voltmeter(Sgnd) 1 ==
  Ground10 : powerlib/Elements/Ground  LConnTagsString=a
  RMS1 : powerlib_meascontrol/Measurements/RMS  TrueRMS=on  Freq=50  RMSInit=0  Ts=1e-4
  Scope1 : Scope
  Scope2 : Scope
  Voltage Measurement1 : powerlib/Measurements/Voltage Measurement  PhasorSimulation=off  OutputType=Complex  PSBequivalent=0
  V+ : PMIOPort  Port=1  Side=Left
  wires:
  Voltage Measurement1/1 -> Scope2/1, RMS1/1
  RMS1/1 -> Scope1/1
  connections:
  Voltage Measurement1/LConn1 -- V+/RConn1
  Ground10/LConn1 -- Voltage Measurement1/LConn2

== system FLANFIS/Voltmeter(Sgnd) 2 ==
  Ground10 : powerlib/Elements/Ground  LConnTagsString=a
  RMS1 : powerlib_meascontrol/Measurements/RMS  TrueRMS=on  Freq=50  RMSInit=0  Ts=1e-4
  Scope1 : Scope
  Scope2 : Scope
  Voltage Measurement1 : powerlib/Measurements/Voltage Measurement  PhasorSimulation=off  OutputType=Complex  PSBequivalent=0
  V+ : PMIOPort  Port=1  Side=Left
  wires:
  Voltage Measurement1/1 -> Scope2/1, RMS1/1
  RMS1/1 -> Scope1/1
  connections:
  Voltage Measurement1/LConn1 -- V+/RConn1
  Ground10/LConn1 -- Voltage Measurement1/LConn2

== system FLANFIS/Voltmeter(gnd) 1 ==
  ERef11 : fl_lib/Electrical/Electrical Elements/Electrical Reference
  PS-Simulink Converter3 : nesl_utility/PS-Simulink Converter  PhysicalDomain=network_engine_domain  SubClassName=ps_output  LeftPortType=input  RightPortType=output  PseudoPeriodic=off  Frequencies=[]  Unit=1  AffineConversion=off
  Scope2 : Scope
  Voltage Sensor2 : fl_lib/Electrical/Electrical Sensors/Voltage Sensor
  V+ : PMIOPort  Port=1  Side=Left
  wires:
  PS-Simulink Converter3/1 -> Scope2/1
  connections:
  Voltage Sensor2/RConn1 -- PS-Simulink Converter3/LConn1
  Voltage Sensor2/RConn2 -- ERef11/LConn1
  Voltage Sensor2/LConn1 -- V+/RConn1

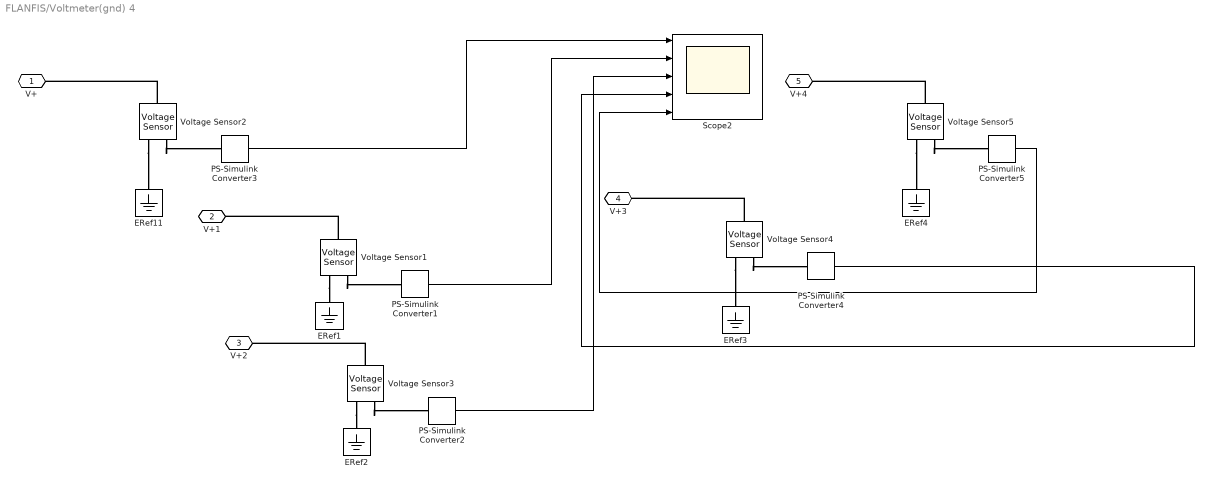
== system FLANFIS/Voltmeter(gnd) 4 ==
  ERef{1..4,11} (5 alike) : fl_lib/Electrical/Electrical Elements/Electrical Reference
  PS-Simulink Converter{1..5} (5 alike) : nesl_utility/PS-Simulink Converter  PhysicalDomain=network_engine_domain  SubClassName=ps_output  LeftPortType=input  RightPortType=output  PseudoPeriodic=off  Frequencies=[]  Unit=1  AffineConversion=off
  Scope2 : Scope  NumInputPorts=5
  Voltage Sensor{1..5} (5 alike) : fl_lib/Electrical/Electrical Sensors/Voltage Sensor
  V+ : PMIOPort  Port=1  Side=Left
  V+1 : PMIOPort  Port=2  Side=Left
  V+2 : PMIOPort  Port=3  Side=Left
  V+3 : PMIOPort  Port=4  Side=Left
  V+4 : PMIOPort  Port=5  Side=Left
  wires:
  PS-Simulink Converter5/1 -> Scope2/5
  PS-Simulink Converter4/1 -> Scope2/4
  PS-Simulink Converter2/1 -> Scope2/3
  PS-Simulink Converter1/1 -> Scope2/2
  PS-Simulink Converter3/1 -> Scope2/1
  connections:
  Voltage Sensor5/RConn2 -- ERef4/LConn1
  Voltage Sensor5/LConn1 -- V+4/RConn1
  Voltage Sensor5/RConn1 -- PS-Simulink Converter5/LConn1
  Voltage Sensor4/RConn1 -- PS-Simulink Converter4/LConn1
  Voltage Sensor4/LConn1 -- V+3/RConn1
  Voltage Sensor4/RConn2 -- ERef3/LConn1
  Voltage Sensor3/RConn2 -- ERef2/LConn1
  Voltage Sensor3/LConn1 -- V+2/RConn1
  Voltage Sensor3/RConn1 -- PS-Simulink Converter2/LConn1
  Voltage Sensor1/RConn1 -- PS-Simulink Converter1/LConn1
  Voltage Sensor1/LConn1 -- V+1/RConn1
  Voltage Sensor1/RConn2 -- ERef1/LConn1
  Voltage Sensor2/LConn1 -- V+/RConn1
  Voltage Sensor2/RConn2 -- ERef11/LConn1
  Voltage Sensor2/RConn1 -- PS-Simulink Converter3/LConn1

== system FLANFIS/Vref ==
  ERef2 : fl_lib/Electrical/Electrical Elements/Electrical Reference
  Vref : elec_lib/Additional Components/SPICE-Compatible Components/Sources/DC Voltage Source  DC=0.78 V
      settings: SourceProductName=Simscape Electronics  SourceProductBaseCode=SN
  Conn1 : PMIOPort  Port=1  Side=Left
  connections:
  Conn1/RConn1 -- Vref/LConn1
  ERef2/LConn1 -- Vref/RConn1
